simulink model "AAI"  (R2022b)
settings: Solver=FixedStepAuto  StartTime=0.0  StopTime=10.0  FixedStep=1e-3  RelTol=1e-3  EnableMultiTasking=on
undefined symbols (not defined in the file): D0, D10, D11, D12, D13, D2, D4, D5, D6, D7, D8, D9, PTA0, PTA2, PTB23, PTB9, PTC16, PTC2, PTC3, PTC4, PTD0, PTD1, PTD2, PTD3
libraries: frdmk64flib x12
settings Model: ExtModeTrigDuration=5  Creator=16475  LastModifiedBy=kaano
settings OptimizationCC: EnhancedBackFolding=on  PassReuseOutputArgsAs=Individual arguments  ZeroExternalMemoryAtStartup=off  ZeroInternalMemoryAtStartup=off  MaxStackSize=64  OptimizeBlockOrder=speed  DifferentSizesBufferReuse=on  OptimizationCustomize=off  EfficientTunableParamExpr=on
settings DebuggingCC: ParameterTunabilityLossMsg=error
settings HardwareCC: ProdBitPerPointer=32  ProdBitPerSizeT=32  ProdBitPerPtrDiffT=32  ProdLargestAtomicInteger=Long  ProdLargestAtomicFloat=Double  ProdWordSize=32  ProdHWDeviceType=ARM Compatible->ARM Cortex
settings SFSimCC: MATLABDynamicMemAlloc=off
settings RTWCC: Description=Embedded Coder  SystemTargetFile=ert.tlc  HardwareBoard=NXP FRDM-K64F  TLCOptions="-aInlineSetEventsForThisBaseRateFcn=TLC_FALSE -aSuppressMultiTaskScheduler=TLC_FALSE  -aRateBasedStepFcn=0"  TemplateMakefile=ert_default_tmf  Toolchain=GNU Tools for ARM Embedded Processors
settings CodeAppCC: ForceParamTrailComments=on  IgnoreCustomStorageClasses=off  OperatorAnnotations=on  SimulinkDataObjDesc=on  SFDataObjDesc=on  InsertBlockDesc=on
settings ERTTargetCC: ExtModeTransport=4  ExtModeMexFile=sendToCommService

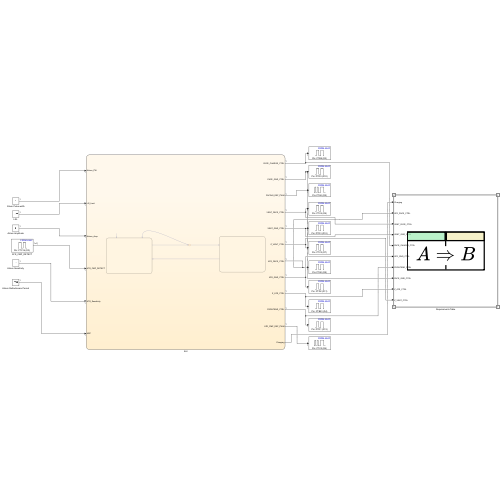
[thumbnail: Simulink's stored preview of the top-level diagram]
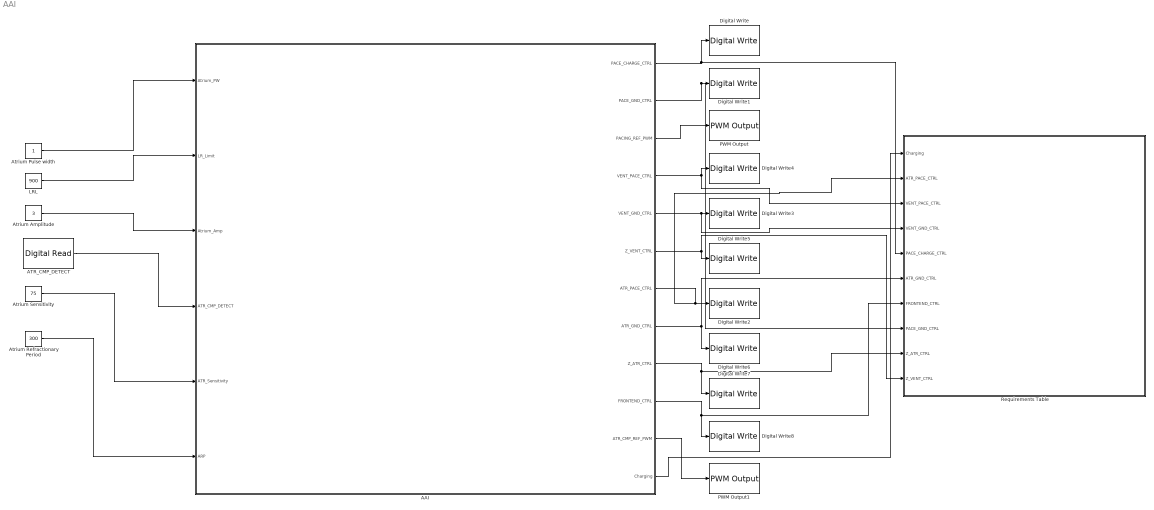
== system AAI ==
  AAI : Stateflow chart  TreatAsAtomicUnit=on
      settings: PortSchema="{\"entries\":[{\"content\":{\"sides\":[{\"content\":{\"connectorIds\":[\"In1\",\"In2\",\"In3\",\"In4\",\"In5\",\"In6\"]},\"type\":\"ConnectorPlacement.EquallySpacedRectSide\",\"uuid\":\"a3e94f58-3093-42a5-91db-f56c9d127bee\"},{\"content\":{\"connectorIds\":[\"Out1\",\"Out2\",\"Out3\",\"Out5\",\"Out4\",\"Out7\",\"Out6\",\"Out8\",\"Out9\",\"Out10\",\"Out11\",\"Out12\"],\"side\":\"RIGHT\"},\"type\":\"ConnectorPlacement.EquallySpacedRectSide\",\"uuid\":\"289ad049-9840-4721-af22-1385d5696f7c\"},{\"content\":{\"connectorIds\":[],\"side\":\"TOP\"},\"type\":\"ConnectorPlacement.EquallySpacedRectSide\",\"uuid\":\"4602f2ad-cb91-4c7a-9db6-6571445db01f\"}]},\"type\":\"ConnectorPlacement.EquallySpacedConnector\",\"uuid\":\"bfd50937-4990-4c1b-ba87-ff4dc7d3240f\"}],\"packageUris\":[\"http://schema.mathworks.com/mf0/Connector/R2020b\"],\"version\":\"1.0\"}"
  ATR_CMP_DETECT : frdmk64flib/Digital Read  Whichpin=PTC16 (D0)  SampleTime=-1
  Atrium Amplitude : Constant  Value=3
  Atrium Pulse width : Constant
  Atrium Refractionary Period : Constant  Value=300
  Atrium Sensitivity : Constant  Value=75
  Digital Write : frdmk64flib/Digital Write  Whichpin=PTB9 (D2)
  Digital Write1 : frdmk64flib/Digital Write  Whichpin=PTD0 (D10)
  Digital Write2 : frdmk64flib/Digital Write  Whichpin=PTA0 (D8)
  Digital Write3 : frdmk64flib/Digital Write  Whichpin=PTD3 (D12)
  Digital Write4 : frdmk64flib/Digital Write  Whichpin=PTC4 (D9)
  Digital Write5 : frdmk64flib/Digital Write  Whichpin=PTC3 (D7)
  Digital Write6 : frdmk64flib/Digital Write  Whichpin=PTD2 (D11)
  Digital Write7 : frdmk64flib/Digital Write  Whichpin=PTB23 (D4)
  Digital Write8 : frdmk64flib/Digital Write  Whichpin=PTD1 (D13)
  LRL : Constant  Value=900
  PWM Output : frdmk64flib/PWM Output  Whichpin=PTA2 (D5)  InitialFrequency=2000  InitialDutyCycle=0
  PWM Output1 : frdmk64flib/PWM Output  Whichpin=PTC2 (D6)  InitialFrequency=2000  InitialDutyCycle=0
  Requirements Table : Requirements Table  TreatAsAtomicUnit=on
  wires:
  AAI/6(ATR_PACE_CTRL) -> Digital Write2/1, Requirements Table/2(ATR_PACE_CTRL)
  AAI/2(PACE_GND_CTRL) -> Requirements Table/8(PACE_GND_CTRL), Digital Write1/1
  LRL/1 -> AAI/2(LR_Limit)
  Atrium Pulse width/1 -> AAI/1(Atrium_PW)
  AAI/4(VENT_GND_CTRL) -> Requirements Table/4(VENT_GND_CTRL), Digital Write3/1
  AAI/9(Z_ATR_CTRL) -> Digital Write7/1, Requirements Table/9(Z_ATR_CTRL)
  Atrium Amplitude/1 -> AAI/3(Atrium_Amp)
  AAI/7(Z_VENT_CTRL) -> Digital Write5/1, Requirements Table/10(Z_VENT_CTRL)
  AAI/3(PACING_REF_PWM) -> PWM Output/1
  AAI/1(PACE_CHARGE_CTRL) -> Digital Write/1, Requirements Table/5(PACE_CHARGE_CTRL)
  AAI/8(ATR_GND_CTRL) -> Digital Write6/1, Requirements Table/6(ATR_GND_CTRL)
  AAI/5(VENT_PACE_CTRL) -> Digital Write4/1, Requirements Table/3(VENT_PACE_CTRL)
  ATR_CMP_DETECT/1 -> AAI/4(ATR_CMP_DETECT)
  AAI/10(FRONTEND_CTRL) -> Digital Write8/1, Requirements Table/7(FRONTEND_CTRL)
  AAI/11(ATR_CMP_REF_PWM) -> PWM Output1/1
  Atrium Sensitivity/1 -> AAI/5(ATR_Sensitivity)
  Atrium Refractionary Period/1 -> AAI/6(ARP)
  AAI/12(Charging) -> Requirements Table/1(Charging)

== stateflow chart AAI/AAI ==
  state Discharging
    entry:
    PACE_CHARGE_CTRL = false;
    PACE_GND_CTRL = true;
    ATR_PACE_CTRL = true;
    VENT_PACE_CTRL = false;
    Z_ATR_CTRL = false;
    Z_VENT_CTRL = false;
    ATR_GND_CTRL = false;
    VENT_GND_CTRL = false;
    FRONTEND_CTRL = false;
    Charging = false;
  state Charging
    entry:
    ATR_PACE_CTRL = false;
    VENT_PACE_CTRL = false;
    PACING_REF_PWM = ((Atrium_Amp/5)*100);
    PACE_CHARGE_CTRL = true;
    PACE_GND_CTRL = true;
    Z_ATR_CTRL = false;
    Z_VENT_CTRL = false;
    ATR_GND_CTRL = true;
    VENT_GND_CTRL = false;
    FRONTEND_CTRL = true;
    ATR_CMP_REF_PWM = ATR_Sensitivity;
    Charging = true;
  (junction 36) -> Charging [order 2] : [ATR_CMP_DETECT == true]
  (default) -> Charging
  Charging -> (junction 36) : [after(ARP,msec)]
  (junction 36) -> Discharging [order 1] : [after(LR_Limit - ARP,msec)]
  Discharging -> Charging : [after(Atrium_PW,msec)]
  data: Atrium_PW input double; LR_Limit input double; PACE_CHARGE_CTRL output boolean; PACE_GND_CTRL output boolean; PACING_REF_PWM output double; VENT_GND_CTRL output boolean; VENT_PACE_CTRL output boolean; ATR_PACE_CTRL output boolean; Z_VENT_CTRL output boolean; Atrium_Amp input double; ATR_GND_CTRL output boolean; Z_ATR_CTRL output boolean; ATR_CMP_DETECT input boolean; FRONTEND_CTRL output boolean; ATR_CMP_REF_PWM output double; ATR_Sensitivity input double; ARP input double; Charging output

== stateflow chart AAI/Requirements Table ==
  (default) -> (junction 1073741860)
  (junction 1073741860) -> (junction 1073741861) : {
      | % SF_REQ_REV_07
      | }
  (junction 1073741861) -> (junction 1073741863) : {
      | % HEADER_ASSIGNMENTS
      |
      | }
  (junction 1073741863) -> (junction 1073741865) : {
      | % START_A_4
      | }
  (junction 1073741865) -> (junction 1073741867) : {
      | }
  (junction 1073741867) -> (junction 1073741869)
  (junction 1073741869) -> (junction 1073741871) : {
      | }
  (junction 1073741871) -> (junction 1073741873) : {
      | % END_A_4
      | }
  (junction 1073741873) -> (junction 1073741922) : {
      | % START_R_1
      | }
  (junction 1073741922) -> (junction 1073741924) : {
      | }
  (junction 1073741924) -> (junction 1073741926)
  (junction 1073741926) -> (junction 1073741928) [order 1] : [(((prev(Charging)) == (prev(Charging) == false)))]
  (junction 1073741926) -> (junction 1073741934) [order 2]
  (junction 1073741928) -> (junction 1073741930) : {
      | reqtable_postcondition((((ATR_PACE_CTRL ) == (false))) && (((VENT_PACE_CTRL ) == (false))) && (((PACE_CHARGE_CTRL ) == (true))) && (((PACE_GND_CTRL ) == (true))) && (((Z_ATR_CTRL ) == (false))) && (((Z_VENT_CTRL ) == (false))) && (((ATR_GND_CTRL ) == (true))) && (((VENT_GND_CTRL ) == (false))) && (((Charging) == (false))) && (((FRONTEND_CTRL ) == (true))), 'R:1');
      |
      |
      | }
  (junction 1073741930) -> (junction 1073741932) : {
      | }
  (junction 1073741932) -> (junction 1073741934)
  (junction 1073741934) -> (junction 1073741936)
  (junction 1073741936) -> (junction 1073741938) : {
      | % END_R_1
      | }
  (junction 1073741938) -> (junction 1073741943) : {
      | % START_R_7
      | }
  (junction 1073741943) -> (junction 1073741945) : {
      | }
  (junction 1073741945) -> (junction 1073741947)
  (junction 1073741947) -> (junction 1073741949) [order 1] : [(((prev(Charging)) == (prev(Charging) == true)))]
  (junction 1073741947) -> (junction 1073741955) [order 2]
  (junction 1073741949) -> (junction 1073741951) : {
      | reqtable_postcondition((((ATR_PACE_CTRL ) == (false))) && (((VENT_PACE_CTRL ) == (true))) && (((PACE_CHARGE_CTRL ) == (true))) && (((PACE_GND_CTRL ) == (false))) && (((Z_ATR_CTRL ) == (false))) && (((Z_VENT_CTRL ) == (false))) && (((ATR_GND_CTRL ) == (false))) && (((VENT_GND_CTRL ) == (false))) && (((Charging) == (true))) && (((FRONTEND_CTRL ) == (false))), 'R:2');
      |
      |
      | }
  (junction 1073741951) -> (junction 1073741953) : {
      | }
  (junction 1073741953) -> (junction 1073741955)
  (junction 1073741955) -> (junction 1073741957)
  (junction 1073741957) -> (junction 1073741959) : {
      | % END_R_7
      | }
  data: Charging input; ATR_PACE_CTRL input; VENT_PACE_CTRL input; VENT_GND_CTRL input; PACE_CHARGE_CTRL input; ATR_GND_CTRL input; FRONTEND_CTRL input; PACE_GND_CTRL input; Z_ATR_CTRL input; Z_VENT_CTRL input
